simulink model "AOO_VOO"  (R2020a)
settings: Solver=FixedStepAuto  StartTime=0.0  StopTime=10.0  FixedStep=1e-3  RelTol=1e-3  EnableMultiTasking=on
settings Model: ExtModeTrigDuration=5  Creator=WinnieTrandinh  LastModifiedBy=WinnieTrandinh
settings OptimizationCC: EnhancedBackFolding=on  PassReuseOutputArgsAs=Individual arguments  ZeroExternalMemoryAtStartup=off  ZeroInternalMemoryAtStartup=off  MaxStackSize=64  OptimizeBlockOrder=speed  DifferentSizesBufferReuse=on  OptimizationCustomize=off  EfficientTunableParamExpr=on
settings DebuggingCC: ParameterTunabilityLossMsg=error
settings HardwareCC: ProdBitPerPointer=32  ProdBitPerSizeT=32  ProdBitPerPtrDiffT=32  ProdLargestAtomicInteger=Long  ProdLargestAtomicFloat=Double  ProdWordSize=32  ProdHWDeviceType=ARM Compatible->ARM Cortex
settings SFSimCC: MATLABDynamicMemAlloc=off
settings RTWCC: SystemTargetFile=ert.tlc  HardwareBoard=NXP FRDM-K64F  TemplateMakefile=ert_default_tmf  Toolchain=GNU Tools for ARM Embedded Processors
settings CodeAppCC: ForceParamTrailComments=on  IgnoreCustomStorageClasses=off  OperatorAnnotations=on  SimulinkDataObjDesc=on  SFDataObjDesc=on  InsertBlockDesc=on

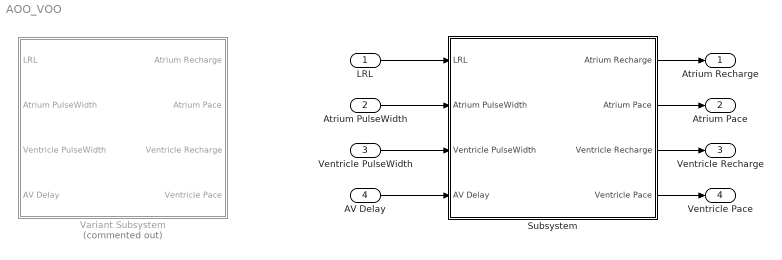
== system AOO_VOO ==
  LRL : Inport
  Atrium PulseWidth : Inport  Port=2
  Ventricle PulseWidth : Inport  Port=3
  AV Delay : Inport  Port=4
  Subsystem : Subsystem
  Variant Subsystem : Subsystem  Commented=on  Variant=on
  Atrium Recharge : Outport
  Atrium Pace : Outport  Port=2
  Ventricle Recharge : Outport  Port=3
  Ventricle Pace : Outport  Port=4
  wires:
  LRL/1 -> Subsystem/1(LRL)
  Atrium PulseWidth/1 -> Subsystem/2(Atrium PulseWidth)
  Subsystem/3(Ventricle Recharge) -> Ventricle Recharge/1
  Subsystem/2(Atrium Pace) -> Atrium Pace/1
  Subsystem/1(Atrium Recharge) -> Atrium Recharge/1
  Subsystem/4(Ventricle Pace) -> Ventricle Pace/1
  Ventricle PulseWidth/1 -> Subsystem/3(Ventricle PulseWidth)
  AV Delay/1 -> Subsystem/4(AV Delay)

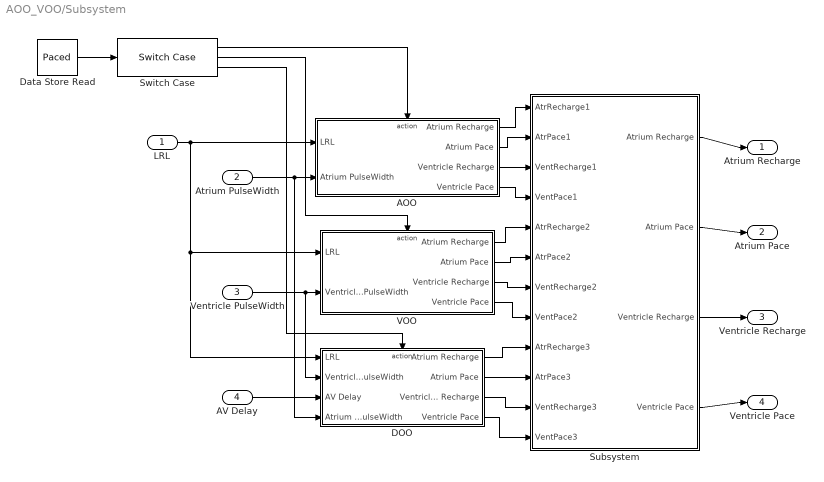
== system AOO_VOO/Subsystem ==
  LRL : Inport
  Atrium PulseWidth : Inport  Port=2
  Ventricle PulseWidth : Inport  Port=3
  AV Delay : Inport  Port=4
  AOO : Subsystem  VariantControl=ATR_PACING
  DOO : Subsystem  VariantControl=DUAL_PACING
  Data Store Read : DataStoreRead  DataStoreName=Paced
  Subsystem : Subsystem
  Switch Case : SwitchCase  CaseConditions={1,2,3}  ShowDefaultCase=off
  VOO : Subsystem  VariantControl=VENT_PACING
  Atrium Recharge : Outport
  Atrium Pace : Outport  Port=2
  Ventricle Recharge : Outport  Port=3
  Ventricle Pace : Outport  Port=4
  wires:
  LRL/1 -> AOO/1(LRL), VOO/1(LRL), DOO/1(LRL)
  Atrium PulseWidth/1 -> AOO/2(Atrium PulseWidth), DOO/4(Atrium PulseWidth)
  Ventricle PulseWidth/1 -> VOO/2(Ventricle PulseWidth), DOO/2(Ventricle PulseWidth)
  AV Delay/1 -> DOO/3(AV Delay)
  AOO/1(Atrium Recharge) -> Subsystem/1(AtrRecharge1)
  AOO/2(Atrium Pace) -> Subsystem/2(AtrPace1)
  AOO/3(Ventricle Recharge) -> Subsystem/3(VentRecharge1)
  AOO/4(Ventricle Pace) -> Subsystem/4(VentPace1)
  VOO/1(Atrium Recharge) -> Subsystem/5(AtrRecharge2)
  VOO/2(Atrium Pace) -> Subsystem/6(AtrPace2)
  VOO/3(Ventricle Recharge) -> Subsystem/7(VentRecharge2)
  VOO/4(Ventricle Pace) -> Subsystem/8(VentPace2)
  DOO/1(Atrium Recharge) -> Subsystem/9(AtrRecharge3)
  DOO/2(Atrium Pace) -> Subsystem/10(AtrPace3)
  DOO/3(Ventricle Recharge) -> Subsystem/11(VentRecharge3)
  DOO/4(Ventricle Pace) -> Subsystem/12(VentPace3)
  Subsystem/4(Ventricle Pace) -> Ventricle Pace/1
  Subsystem/1(Atrium Recharge) -> Atrium Recharge/1
  Subsystem/2(Atrium Pace) -> Atrium Pace/1
  Subsystem/3(Ventricle Recharge) -> Ventricle Recharge/1
  Data Store Read/1 -> Switch Case/1
  Switch Case/1 -> AOO/Action
  Switch Case/2 -> VOO/Action
  Switch Case/3 -> DOO/Action

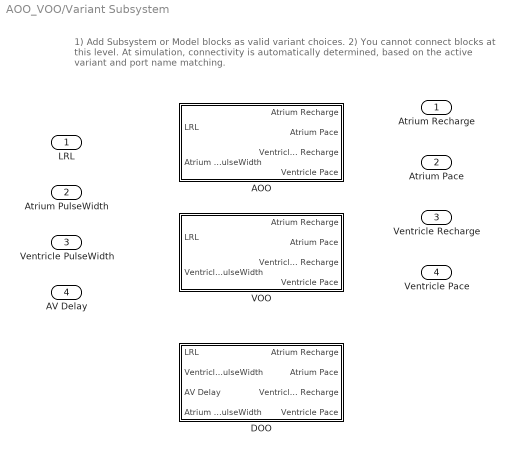
== system AOO_VOO/Variant Subsystem ==
  note: 1) Add Subsystem or Model blocks as valid variant choices.
      | 2) You cannot connect blocks at this level. At simulation, connectivity is automatically
      | determined, based on the active variant and port name matching.
  LRL : Inport
  Atrium PulseWidth : Inport  Port=2
  Ventricle PulseWidth : Inport  Port=3
  AV Delay : Inport  Port=4
  AOO : Subsystem  VariantControl=ATR_PACING
  DOO : Subsystem  VariantControl=DUAL_PACING
  VOO : Subsystem  VariantControl=VENT_PACING
  Atrium Recharge : Outport
  Atrium Pace : Outport  Port=2
  Ventricle Recharge : Outport  Port=3
  Ventricle Pace : Outport  Port=4

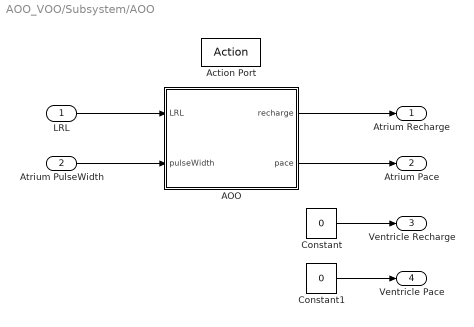
== system AOO_VOO/Subsystem/AOO ==
  LRL : Inport
  Atrium PulseWidth : Inport  Port=2
  Action Port : ActionPort  ActionPortLabel=case [ 1 ]:
  AOO : Stateflow chart  TreatAsAtomicUnit=on
  Constant : Constant  Value=0
  Constant1 : Constant  Value=0  OutDataTypeStr=boolean
  Atrium Recharge : Outport
  Atrium Pace : Outport  Port=2
  Ventricle Recharge : Outport  Port=3
  Ventricle Pace : Outport  Port=4
  wires:
  LRL/1 -> AOO/1(LRL)
  Atrium PulseWidth/1 -> AOO/2(pulseWidth)
  AOO/1(recharge) -> Atrium Recharge/1
  AOO/2(pace) -> Atrium Pace/1
  Constant/1 -> Ventricle Recharge/1
  Constant1/1 -> Ventricle Pace/1

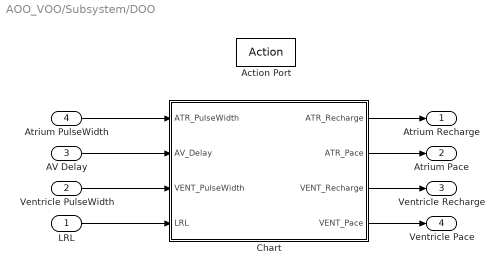
== system AOO_VOO/Subsystem/DOO ==
  LRL : Inport
  Ventricle PulseWidth : Inport  Port=2
  AV Delay : Inport  Port=3
  Atrium PulseWidth : Inport  Port=4
  Action Port : ActionPort  ActionPortLabel=case [ 3 ]:
  Chart : Stateflow chart  TreatAsAtomicUnit=on
  Atrium Recharge : Outport
  Atrium Pace : Outport  Port=2
  Ventricle Recharge : Outport  Port=3
  Ventricle Pace : Outport  Port=4
  wires:
  Chart/2(ATR_Pace) -> Atrium Pace/1
  Chart/1(ATR_Recharge) -> Atrium Recharge/1
  Chart/4(VENT_Pace) -> Ventricle Pace/1
  Ventricle PulseWidth/1 -> Chart/3(VENT_PulseWidth)
  LRL/1 -> Chart/4(LRL)
  Chart/3(VENT_Recharge) -> Ventricle Recharge/1
  Atrium PulseWidth/1 -> Chart/1(ATR_PulseWidth)
  AV Delay/1 -> Chart/2(AV_Delay)

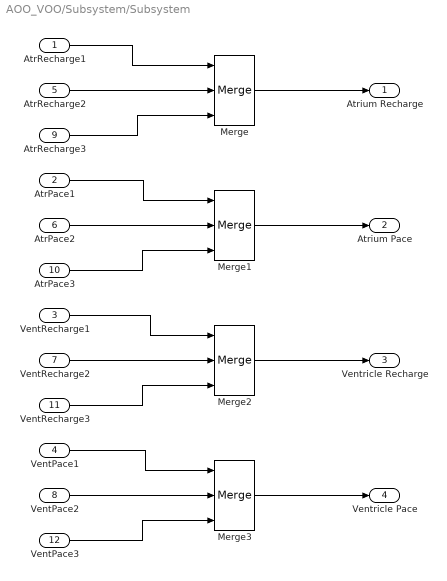
== system AOO_VOO/Subsystem/Subsystem ==
  AtrRecharge1 : Inport
  AtrPace1 : Inport  Port=2
  VentRecharge1 : Inport  Port=3
  VentPace1 : Inport  Port=4
  AtrRecharge2 : Inport  Port=5
  AtrPace2 : Inport  Port=6
  VentRecharge2 : Inport  Port=7
  VentPace2 : Inport  Port=8
  AtrRecharge3 : Inport  Port=9
  AtrPace3 : Inport  Port=10
  VentRecharge3 : Inport  Port=11
  VentPace3 : Inport  Port=12
  Merge{,1..3} (4 alike) : Merge  Inputs=3
  Atrium Recharge : Outport
  Atrium Pace : Outport  Port=2
  Ventricle Recharge : Outport  Port=3
  Ventricle Pace : Outport  Port=4
  wires:
  AtrRecharge2/1 -> Merge/2
  AtrRecharge1/1 -> Merge/1
  AtrRecharge3/1 -> Merge/3
  Merge/1 -> Atrium Recharge/1
  AtrPace2/1 -> Merge1/2
  AtrPace1/1 -> Merge1/1
  AtrPace3/1 -> Merge1/3
  Merge1/1 -> Atrium Pace/1
  VentRecharge2/1 -> Merge2/2
  VentRecharge1/1 -> Merge2/1
  VentRecharge3/1 -> Merge2/3
  Merge2/1 -> Ventricle Recharge/1
  VentPace1/1 -> Merge3/1
  VentPace2/1 -> Merge3/2
  VentPace3/1 -> Merge3/3
  Merge3/1 -> Ventricle Pace/1

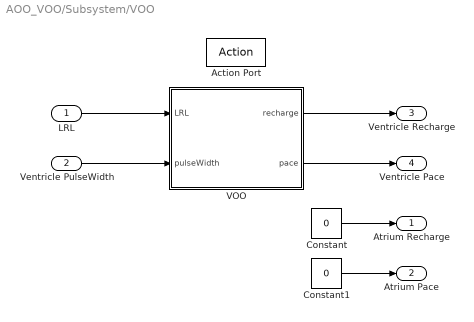
== system AOO_VOO/Subsystem/VOO ==
  LRL : Inport
  Ventricle PulseWidth : Inport  Port=2
  Action Port : ActionPort  ActionPortLabel=case [ 2 ]:
  Constant : Constant  Value=0
  Constant1 : Constant  Value=0  OutDataTypeStr=boolean
  VOO : Stateflow chart  TreatAsAtomicUnit=on
  Atrium Recharge : Outport
  Atrium Pace : Outport  Port=2
  Ventricle Recharge : Outport  Port=3
  Ventricle Pace : Outport  Port=4
  wires:
  LRL/1 -> VOO/1(LRL)
  Ventricle PulseWidth/1 -> VOO/2(pulseWidth)
  VOO/1(recharge) -> Ventricle Recharge/1
  VOO/2(pace) -> Ventricle Pace/1
  Constant/1 -> Atrium Recharge/1
  Constant1/1 -> Atrium Pace/1

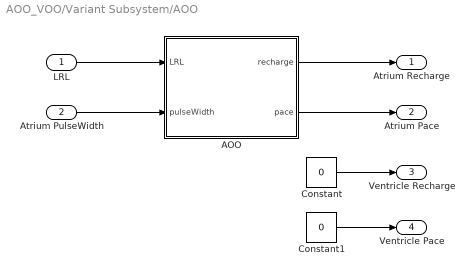
== system AOO_VOO/Variant Subsystem/AOO ==
  LRL : Inport
  Atrium PulseWidth : Inport  Port=2
  AOO : Stateflow chart  TreatAsAtomicUnit=on
  Constant : Constant  Value=0
  Constant1 : Constant  Value=0  OutDataTypeStr=boolean
  Atrium Recharge : Outport
  Atrium Pace : Outport  Port=2
  Ventricle Recharge : Outport  Port=3
  Ventricle Pace : Outport  Port=4
  wires:
  LRL/1 -> AOO/1(LRL)
  Atrium PulseWidth/1 -> AOO/2(pulseWidth)
  AOO/1(recharge) -> Atrium Recharge/1
  AOO/2(pace) -> Atrium Pace/1
  Constant/1 -> Ventricle Recharge/1
  Constant1/1 -> Ventricle Pace/1

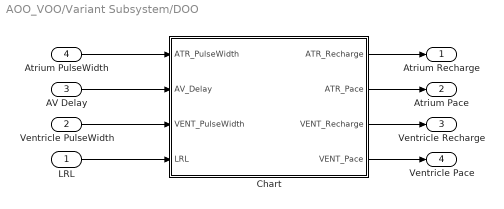
== system AOO_VOO/Variant Subsystem/DOO ==
  LRL : Inport
  Ventricle PulseWidth : Inport  Port=2
  AV Delay : Inport  Port=3
  Atrium PulseWidth : Inport  Port=4
  Chart : Stateflow chart  TreatAsAtomicUnit=on
  Atrium Recharge : Outport
  Atrium Pace : Outport  Port=2
  Ventricle Recharge : Outport  Port=3
  Ventricle Pace : Outport  Port=4
  wires:
  Chart/2(ATR_Pace) -> Atrium Pace/1
  Chart/1(ATR_Recharge) -> Atrium Recharge/1
  Chart/4(VENT_Pace) -> Ventricle Pace/1
  Ventricle PulseWidth/1 -> Chart/3(VENT_PulseWidth)
  LRL/1 -> Chart/4(LRL)
  Chart/3(VENT_Recharge) -> Ventricle Recharge/1
  Atrium PulseWidth/1 -> Chart/1(ATR_PulseWidth)
  AV Delay/1 -> Chart/2(AV_Delay)

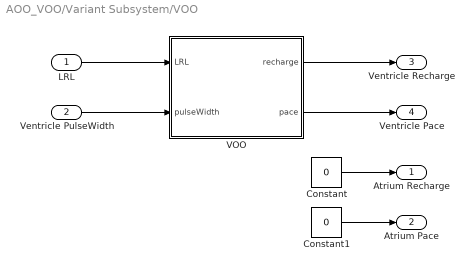
== system AOO_VOO/Variant Subsystem/VOO ==
  LRL : Inport
  Ventricle PulseWidth : Inport  Port=2
  Constant : Constant  Value=0
  Constant1 : Constant  Value=0  OutDataTypeStr=boolean
  VOO : Stateflow chart  TreatAsAtomicUnit=on
  Atrium Recharge : Outport
  Atrium Pace : Outport  Port=2
  Ventricle Recharge : Outport  Port=3
  Ventricle Pace : Outport  Port=4
  wires:
  LRL/1 -> VOO/1(LRL)
  Ventricle PulseWidth/1 -> VOO/2(pulseWidth)
  VOO/1(recharge) -> Ventricle Recharge/1
  VOO/2(pace) -> Ventricle Pace/1
  Constant/1 -> Atrium Recharge/1
  Constant1/1 -> Atrium Pace/1

== stateflow chart AOO_VOO/Subsystem/DOO/Chart ==
  state ATR_Recharge
    entry:
    ATR_Recharge=2;
  state ATR_Recharge_init
    entry:
    ATR_Pace=false;
    VENT_Pace=false;
    ATR_Recharge=1;
  state ATR_Pace
    entry:
    ATR_Pace=true;
    ATR_Recharge=0;
  state VENT_Recharge_init
    entry:
    ATR_Pace=false;
    VENT_Pace=false;
    VENT_Recharge=1;
  state VENT_Pace
    entry:
    VENT_Pace=true;
    VENT_Recharge=0;
  state VENT_Recharge
    entry:
    VENT_Recharge=2;
  (default) -> ATR_Recharge_init
  ATR_Recharge_init -> ATR_Recharge
  ATR_Recharge -> ATR_Pace : [after(LRL-ATR_PulseWidth-VENT_PulseWidth-AV_Delay,msec)]
  ATR_Pace -> VENT_Recharge_init : [after(ATR_PulseWidth,msec)]
  VENT_Pace -> ATR_Recharge_init : [after(VENT_PulseWidth,msec)]
  VENT_Recharge_init -> VENT_Recharge
  VENT_Recharge -> VENT_Pace : [after(AV_Delay,msec)]
  data: ATR_PulseWidth input; AV_Delay input; VENT_PulseWidth input; ATR_Recharge output; ATR_Pace output; VENT_Recharge output; VENT_Pace output; LRL input

== stateflow chart AOO_VOO/Subsystem/VOO/VOO ==
  state Recharge_Init
    entry:
    pace = false;
    recharge = 1;
  note: Sets up for charging C22
      | and discharging C21.
  note: Recharge phase split into two to
      | ensure correct pin activation order.
  state Pace
    entry:
    pace = true;
    recharge = 0;
  state Recharge
    entry:
    recharge = 2;
  note: Starts charging of C22
      | and discharging of C21.
  note: Paces the heart by discharging
      | C22 into the heart.
  (default) -> Recharge_Init
  Pace -> Recharge_Init : [after(pulseWidth, msec)]
  Recharge_Init -> Recharge
  Recharge -> Pace : [after(LRL, msec)]
  data: recharge output; pace output; LRL input; pulseWidth input

== stateflow chart AOO_VOO/Variant Subsystem/VOO/VOO ==
  state Recharge_Init
    entry:
    pace = false;
    recharge = 1;
  note: Sets up for charging C22
      | and discharging C21.
  note: Recharge phase split into two to
      | ensure correct pin activation order.
  state Pace
    entry:
    pace = true;
    recharge = 0;
  state Recharge
    entry:
    recharge = 2;
  note: Starts charging of C22
      | and discharging of C21.
  note: Paces the heart by discharging
      | C22 into the heart.
  (default) -> Recharge_Init
  Pace -> Recharge_Init : [after(pulseWidth, msec)]
  Recharge_Init -> Recharge
  Recharge -> Pace : [after(LRL, msec)]
  data: recharge output; pace output; LRL input; pulseWidth input

== stateflow chart AOO_VOO/Variant Subsystem/DOO/Chart ==
  state ATR_Recharge
    entry:
    ATR_Recharge=2;
  state ATR_Recharge_init
    entry:
    ATR_Pace=false;
    VENT_Pace=false;
    ATR_Recharge=1;
  state ATR_Pace
    entry:
    ATR_Pace=true;
    ATR_Recharge=0;
  state VENT_Recharge_init
    entry:
    ATR_Pace=false;
    VENT_Pace=false;
    VENT_Recharge=1;
  state VENT_Pace
    entry:
    VENT_Pace=true;
    VENT_Recharge=0;
  state VENT_Recharge
    entry:
    VENT_Recharge=2;
  (default) -> ATR_Recharge_init
  ATR_Recharge_init -> ATR_Recharge
  ATR_Recharge -> ATR_Pace : [after(LRL-ATR_PulseWidth-VENT_PulseWidth-AV_Delay,msec)]
  ATR_Pace -> VENT_Recharge_init : [after(ATR_PulseWidth,msec)]
  VENT_Pace -> ATR_Recharge_init : [after(VENT_PulseWidth,msec)]
  VENT_Recharge_init -> VENT_Recharge
  VENT_Recharge -> VENT_Pace : [after(AV_Delay,msec)]
  data: ATR_PulseWidth input; AV_Delay input; VENT_PulseWidth input; ATR_Recharge output; ATR_Pace output; VENT_Recharge output; VENT_Pace output; LRL input

== stateflow chart AOO_VOO/Variant Subsystem/AOO/AOO ==
  state Recharge_Init
    entry:
    pace = false;
    recharge = 1;
  note: Sets up for charging C22
      | and discharging C21.
  note: Recharge phase split into two to
      | ensure correct pin activation order.
  state Pace
    entry:
    pace = true;
    recharge = 0;
  state Recharge
    entry:
    recharge = 2;
  note: Starts charging of C22
      | and discharging of C21.
  note: Paces the heart by discharging
      | C22 into the heart.
  (default) -> Recharge_Init
  Pace -> Recharge_Init : [after(pulseWidth, msec)]
  Recharge_Init -> Recharge
  Recharge -> Pace : [after(LRL, msec)]
  data: recharge output; pace output; LRL input; pulseWidth input

== stateflow chart AOO_VOO/Subsystem/AOO/AOO ==
  state Recharge_Init
    entry:
    pace = false;
    recharge = 1;
  note: Sets up for charging C22
      | and discharging C21.
  note: Recharge phase split into two to
      | ensure correct pin activation order.
  state Pace
    entry:
    pace = true;
    recharge = 0;
  state Recharge
    entry:
    recharge = 2;
  note: Starts charging of C22
      | and discharging of C21.
  note: Paces the heart by discharging
      | C22 into the heart.
  (default) -> Recharge_Init
  Pace -> Recharge_Init : [after(pulseWidth, msec)]
  Recharge_Init -> Recharge
  Recharge -> Pace : [after(LRL, msec)]
  data: recharge output; pace output; LRL input; pulseWidth input
